simulink model "c2837xd_ipc_cpu1_tx"  (R2021b)
settings: Solver=FixedStepDiscrete  StartTime=0.0  StopTime=inf  RelTol=1e-3  EnableMultiTasking=on
undefined symbols (not defined in the file or in its folder): C28x, CPU1, CPU2
libraries: c2837xDlib x4, demo_controls x1, simulink x1
settings Model: ExtModeTrigDuration=8  Creator=The MathWorks, Inc.  LastModifiedBy=The MathWorks, Inc.
settings SolverCC: AlgebraicLoopSolver=TrustRegion  MinimalZcImpactIntegration=on
settings DataIOCC: ReturnWorkspaceOutputs=off
settings OptimizationCC: DefaultUnderspecifiedDataType=single  EnhancedBackFolding=on  StrengthReduction=on  PassReuseOutputArgsAs=Individual arguments  MaxStackSize=512  OptimizeBlockOrder=speed  DifferentSizesBufferReuse=on  EfficientTunableParamExpr=on
settings DebuggingCC: ParameterPrecisionLossMsg=none  ParameterTunabilityLossMsg=error  SFMachineParentedDataDiag=warning  ArithmeticOperatorsInVariantConditions=warning
settings HardwareCC: ProdBitPerChar=16  ProdBitPerInt=16  ProdBitPerPointer=32  ProdBitPerSizeT=32  ProdBitPerPtrDiffT=32  ProdLargestAtomicInteger=Integer  ProdLargestAtomicFloat=None  ProdWordSize=16  ProdLongLongMode=on  ProdHWDeviceType=Texas Instruments->C2000
settings SFSimCC: SimUseLocalCustomCode=off  MATLABDynamicMemAlloc=off  CustomCodeUndefinedFunction=UseInterfaceOnly
settings RTWCC: Description=Embedded Coder  SystemTargetFile=ert.tlc  HardwareBoard=TI Delfino F2837xD  TemplateMakefile=ert_default_tmf  GenerateReport=on  RTWUseLocalCustomCode=off  Toolchain=Texas Instruments Code Composer Studio (C2000)  BuildConfiguration=Debug  IncludeHyperlinkInReport=on  LaunchReport=on  GenerateTraceInfo=on  GenerateTraceReport=on  GenerateTraceReportSl=on  GenerateTraceReportSf=on  GenerateTraceReportEml=on
settings CodeAppCC: ForceParamTrailComments=on  IgnoreCustomStorageClasses=off  OperatorAnnotations=on  SimulinkDataObjDesc=on  SFDataObjDesc=on  InsertBlockDesc=on
settings ERTTargetCC: CodeReplacementLibrary=TI C28x  ExtModeTransport=4  ExtModeStaticAlloc=on  ExtModeStaticAllocSize=10000  ExtModeMexFile=ext_xcp  ExtModeIntrfLevel=Level2 - Open

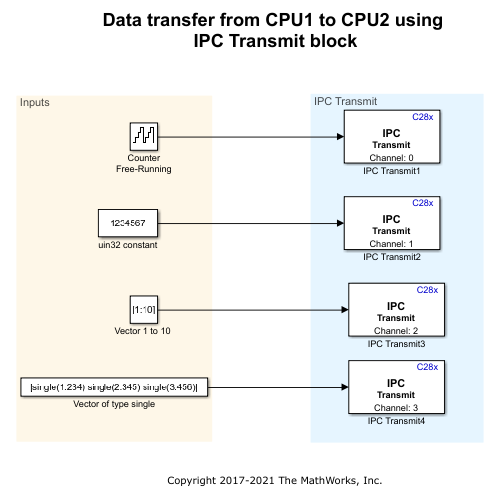
[thumbnail: Simulink's stored preview of the top-level diagram]
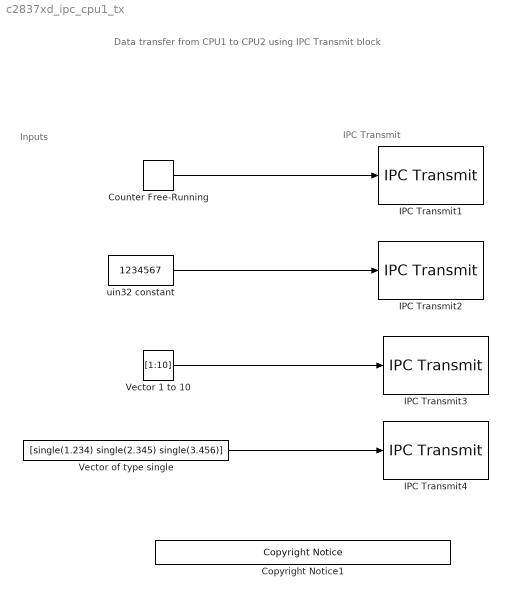
== system c2837xd_ipc_cpu1_tx ==
  note: IPC Transmit
  note: Inputs
  note: Data transfer from CPU1 to CPU2 using
      | IPC Transmit block
  Copyright Notice1 : demo_controls/Copyright Notice  year=2017  prod=tic2000
      settings: SourceProductBaseCode=ME
  Counter Free-Running : simulink/Sources/Counter Free-Running  NumBits=16  tsamp=1
  IPC Transmit1 : c2837xDlib/IPC Transmit  blkParamProc=F2837x  SelectDestination=C28x (CPU1/CPU2)  SelectChannel=0  EnableBlocking=off
      settings: SourceProductBaseCode=TIC2000
  IPC Transmit2 : c2837xDlib/IPC Transmit  blkParamProc=F2837x  SelectDestination=C28x (CPU1/CPU2)  SelectChannel=1  EnableBlocking=off
      settings: SourceProductBaseCode=TIC2000
  IPC Transmit3 : c2837xDlib/IPC Transmit  blkParamProc=F2837x  SelectDestination=C28x (CPU1/CPU2)  SelectChannel=2  EnableBlocking=off
      settings: SourceProductBaseCode=TIC2000
  IPC Transmit4 : c2837xDlib/IPC Transmit  blkParamProc=F2837x  SelectDestination=C28x (CPU1/CPU2)  SelectChannel=3  EnableBlocking=off
      settings: SourceProductBaseCode=TIC2000
  "Vector 1 to 10 " : Constant  Value=[1:10]  OutDataTypeStr=uint16  SampleTime=0.1
  Vector of type single : Constant  Value=[single(1.234) single(2.345) single(3.456)]  OutDataTypeStr=single  SampleTime=.01
  uin32 constant : Constant  Value=1234567  OutDataTypeStr=uint32  SampleTime=0.5
  wires:
  uin32 constant/1 -> IPC Transmit2/1
  "Vector 1 to 10 "/1 -> IPC Transmit3/1
  Vector of type single/1 -> IPC Transmit4/1
  Counter Free-Running/1 -> IPC Transmit1/1
